simulink subsystem "decoder"  (R2019b)
settings: Solver=VariableStepAuto  StartTime=0.0  StopTime=10.0  RelTol=1e-3
InitFcn:
  | %% DSPBuilder Start
  | alt_dspbuilder_update_model(bdroot)
  | %% DSPBuilder End
StartFcn:
  | %% DSPBuilder Start
  | alt_dspbuilder_hdlimport_prepare_for_simulation(bdroot)
  | %% DSPBuilder End
undefined symbols (not defined in the file or in its folder): state
libraries: allblocks_alteradspbuilder2 x30
settings Model: Creator=vboxuser  LastModifiedBy=vboxuser

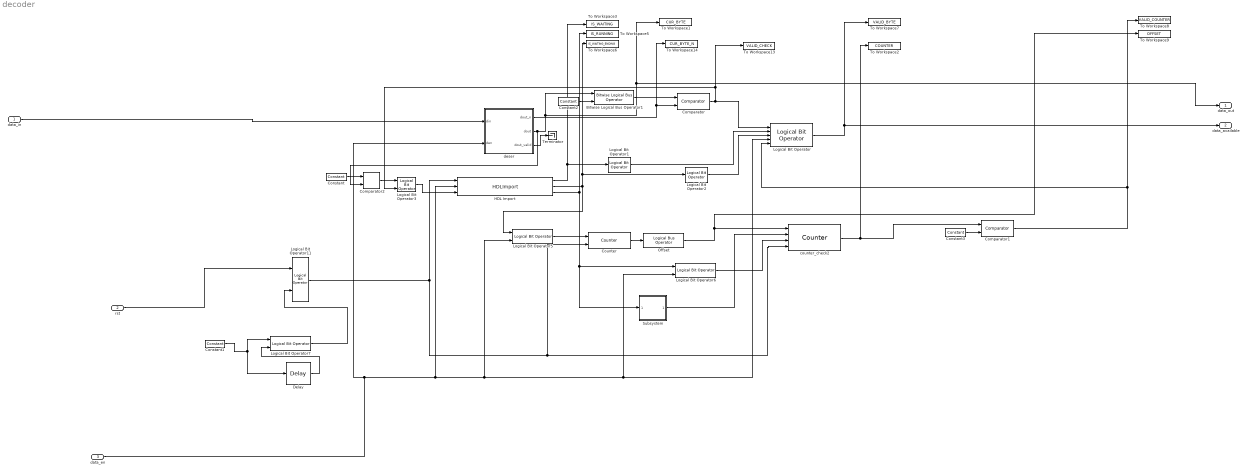
== system decoder ==
  data_in : Inport
  rst : Inport  Port=2
  data_en : Inport  Port=3
  Bitwise Logical Bus Operator1 : allblocks_alteradspbuilder2/Bitwise Logical Bus Operator  BusType=Unsigned Integer  bwl=8  bwr=0  LogicalOperator=XOR  pipeline_display=0
  Comparator : allblocks_alteradspbuilder2/Comparator  direction=a == b  pipeline_display=0  allowFloatingPointOverride=on  logOutputs=off  logFile=C:\Users\vboxuser\Documents\MATLAB\serializer\system2\tb_matcher_simu_old\matcher%5Fsimu%5Fold_Subsystem2_Subsystem_Comparator.fixedpointlog
  Comparator1 : allblocks_alteradspbuilder2/Comparator  direction=a == b  pipeline_display=0  allowFloatingPointOverride=on  logOutputs=off  logFile=C:\Users\vboxuser\Documents\MATLAB\serializer\system2\tb_matcher_simu_old\matcher%5Fsimu%5Fold_Subsystem2_Subsystem_Comparator1.fixedpointlog
  Comparator2 : allblocks_alteradspbuilder2/Comparator  direction=a == b  pipeline_display=0  allowFloatingPointOverride=on  logOutputs=off  logFile=C:\Users\vboxuser\Documents\MATLAB\serializer\system2\tb_matcher_simu_old\matcher%5Fsimu%5Fold_Subsystem2_Subsystem_Comparator2.fixedpointlog
  Constant : allblocks_alteradspbuilder2/Constant  mask_cst=71  BusType=Unsigned Integer  bwl=8  bwr=0  roundMode=Truncate  satMode=Wrap  SpecifyClock=off  allowFloatingPointOverride=on  logOutputs=off  logFile=C:\Users\vboxuser\Documents\MATLAB\serializer\system2\tb_matcher_simu_old\matcher%5Fsimu%5Fold_Subsystem2_Subsystem_Constant.fixedpointlog
  Constant1 : allblocks_alteradspbuilder2/Constant  mask_cst=1  BusType=Single Bit  bwl=8  bwr=0  roundMode=Truncate  satMode=Saturate  SpecifyClock=off  allowFloatingPointOverride=on  logOutputs=off  logFile=C:\Users\vboxuser\Documents\MATLAB\serializer\system2\tb_matcher_simu_old\matcher%5Fsimu%5Fold_Subsystem2_Subsystem_Constant1.fixedpointlog
  Constant2 : allblocks_alteradspbuilder2/Constant  mask_cst=255  BusType=Unsigned Integer  bwl=8  bwr=0  roundMode=Truncate  satMode=Wrap  SpecifyClock=off  allowFloatingPointOverride=on  logOutputs=off  logFile=C:\Users\vboxuser\Documents\MATLAB\serializer\system2\tb_matcher_simu_old\matcher%5Fsimu%5Fold_Subsystem2_Subsystem_Constant2.fixedpointlog
  Constant3 : allblocks_alteradspbuilder2/Constant  mask_cst=159  BusType=Unsigned Integer  bwl=8  bwr=0  roundMode=Truncate  satMode=Saturate  SpecifyClock=off  allowFloatingPointOverride=on  logOutputs=off  logFile=C:\Users\vboxuser\Documents\MATLAB\serializer\system2\tb_matcher_simu_old\matcher%5Fsimu%5Fold_Subsystem2_Subsystem_Constant3.fixedpointlog
  Counter : allblocks_alteradspbuilder2/Counter  BusType=Unsigned Integer  bwl=8  bwr=0  use_modulo=on  modulo=10  SpecifyClock=off  direction=Increment  use_sload=off  use_sset=off  svalue=1  use_clk_ena=off  use_ena=on  use_sclr=on  pipeline_display=1
  Delay : allblocks_alteradspbuilder2/Delay  pipeline=1  pipeline_display=1  ClockPhase=1  use_ena=off  use_sclr=off  allowFloatingPointOverride=on  logOutputs=off  logFile=C:\Users\vboxuser\Documents\MATLAB\serializer\system2\tb_matcher_simu_old\matcher%5Fsimu%5Fold_Subsystem2_Subsystem_Delay.fixedpointlog  use_init=off  reset_value=1
  HDL Import : allblocks_alteradspbuilder2/HDLImport  entityName=state_machine_import  inNames=rst ena is_matching  inBwls=1 1 1  inBwrs="0  0  0"  inTypes=b b b  inDelayed="0  0  0"  outNames=is_waiting is_waiting_ending is_running  outBwls=1 1 1  outBwrs="0  0  0"  outTypes=b b b  xmlmapfile=D:\pliki-programow\intel\18.1\quartus\dsp_builder\lib\SimgenCMap.xml  vofile=DSPBuilder_matcher_simu_import\state_machine.vo  src_file=state.v;  TopLevelName=state_machine  UseQPF=0  n_input_port=3  n_output_port=3  array_clocks=clk  use_systemC_model=off  is_megacore=off  use_dynamic_feedthrough_data=off  use_alphabetical_port_ordering=off  allowFloatingPointOverride=off  id=0  id_is_set=off  UseModelSimBasedFlow=off
  Logical Bit Operator : allblocks_alteradspbuilder2/Logical Bit Operator  LogicalOperator=AND  user_inputs=5  pipeline_display=0
  Logical Bit Operator1 : allblocks_alteradspbuilder2/Logical Bit Operator  LogicalOperator=NOT  user_inputs=2  pipeline_display=0
  Logical Bit Operator11 : allblocks_alteradspbuilder2/Logical Bit Operator  LogicalOperator=OR  user_inputs=2  pipeline_display=0
  Logical Bit Operator2 : allblocks_alteradspbuilder2/Logical Bit Operator  LogicalOperator=NOT  user_inputs=2  pipeline_display=0
  Logical Bit Operator3 : allblocks_alteradspbuilder2/Logical Bit Operator  LogicalOperator=AND  user_inputs=2  pipeline_display=0
  Logical Bit Operator5 : allblocks_alteradspbuilder2/Logical Bit Operator  LogicalOperator=AND  user_inputs=2  pipeline_display=0
  Logical Bit Operator6 : allblocks_alteradspbuilder2/Logical Bit Operator  LogicalOperator=AND  user_inputs=2  pipeline_display=0
  Logical Bit Operator7 : allblocks_alteradspbuilder2/Logical Bit Operator  LogicalOperator=XOR  user_inputs=2  pipeline_display=0
  Offset : allblocks_alteradspbuilder2/Logical Bus Operator  BusType=Unsigned Integer  bwl=8  bwr=0  LogicalOp_text=Shift Right  mask_value_num=-5  shift_amount=1  force_sign_ext=on  pipeline_display=0
  Subsystem : Subsystem  ReferencedSubsystem=Puls
  Terminator : Terminator
  To Workspace1 : ToWorkspace  VariableName=CUR_BYTE  SampleTime=-1
      settings: Save2DSignal=2-D array (concatenate along first dimension)
  To Workspace13 : ToWorkspace  VariableName=VALID_CHECK  SampleTime=-1
      settings: Save2DSignal=2-D array (concatenate along first dimension)
  To Workspace14 : ToWorkspace  VariableName=CUR_BYTE_N  SampleTime=-1
      settings: Save2DSignal=2-D array (concatenate along first dimension)
  To Workspace2 : ToWorkspace  VariableName=COUNTER  SampleTime=-1
      settings: Save2DSignal=2-D array (concatenate along first dimension)
  To Workspace3 : ToWorkspace  VariableName=IS_WAITING  SampleTime=-1
      settings: Save2DSignal=2-D array (concatenate along first dimension)
  To Workspace5 : ToWorkspace  VariableName=IS_RUNNING  SampleTime=-1
      settings: Save2DSignal=2-D array (concatenate along first dimension)
  To Workspace6 : ToWorkspace  VariableName=IS_WAITING_ENDING  SampleTime=-1
      settings: Save2DSignal=2-D array (concatenate along first dimension)
  To Workspace7 : ToWorkspace  VariableName=VALID_BYTE  SampleTime=-1
      settings: Save2DSignal=2-D array (concatenate along first dimension)
  To Workspace8 : ToWorkspace  VariableName=VALID_COUNTER  SampleTime=-1
      settings: Save2DSignal=2-D array (concatenate along first dimension)
  To Workspace9 : ToWorkspace  VariableName=OFFSET  SampleTime=-1
      settings: Save2DSignal=2-D array (concatenate along first dimension)
  counter_check2 : allblocks_alteradspbuilder2/Counter  BusType=Unsigned Integer  bwl=8  bwr=0  use_modulo=on  modulo=160  SpecifyClock=off  direction=Increment  use_sload=on  use_sset=off  svalue=1  use_clk_ena=off  use_ena=on  use_sclr=on  pipeline_display=1
  deser : Subsystem
  data_out : Outport
  data_available : Outport  Port=2
  wires:
  Subsystem/1 -> counter_check2/2
  rst/1 -> Logical Bit Operator11/1
  data_in/1 -> deser/1(din)
  Logical Bit Operator11/1 -> Counter/2, counter_check2/4, HDL Import/1
  deser/3(dout_valid) -> Terminator/1
  Logical Bit Operator7/1 -> Logical Bit Operator11/2
  Delay/1 -> Logical Bit Operator7/2
  Constant1/1 -> Logical Bit Operator7/1, Delay/1
  Logical Bit Operator6/1 -> counter_check2/3
  Counter/1 -> Offset/1
  Constant2/1 -> Bitwise Logical Bus Operator1/2
  Bitwise Logical Bus Operator1/1 -> Comparator/1
  Offset/1 -> To Workspace9/1, counter_check2/1
  Logical Bit Operator1/1 -> Logical Bit Operator/2
  Logical Bit Operator/1 -> data_available/1, To Workspace7/1
  HDL Import/1 -> To Workspace3/1, Logical Bit Operator1/1
  Constant3/1 -> Comparator1/2
  Comparator/1 -> Logical Bit Operator/1, To Workspace13/1, Logical Bit Operator3/2
  HDL Import/3 -> Subsystem/1, Logical Bit Operator6/1, To Workspace5/1
  Comparator1/1 -> Logical Bit Operator/5, To Workspace8/1
  deser/2(dout) -> data_out/1, To Workspace1/1, Bitwise Logical Bus Operator1/1, Comparator2/2
  Logical Bit Operator3/1 -> HDL Import/3
  deser/1(dout_n) -> To Workspace14/1, Comparator/2
  HDL Import/2 -> To Workspace6/1, Logical Bit Operator2/1, Logical Bit Operator5/1
  data_en/1 -> Logical Bit Operator5/2, Logical Bit Operator6/2, Logical Bit Operator/4, HDL Import/2, deser/2(den)
  counter_check2/1 -> To Workspace2/1, Comparator1/1
  Logical Bit Operator2/1 -> Logical Bit Operator/3
  Logical Bit Operator5/1 -> Counter/1
  Constant/1 -> Comparator2/1
  Comparator2/1 -> Logical Bit Operator3/1

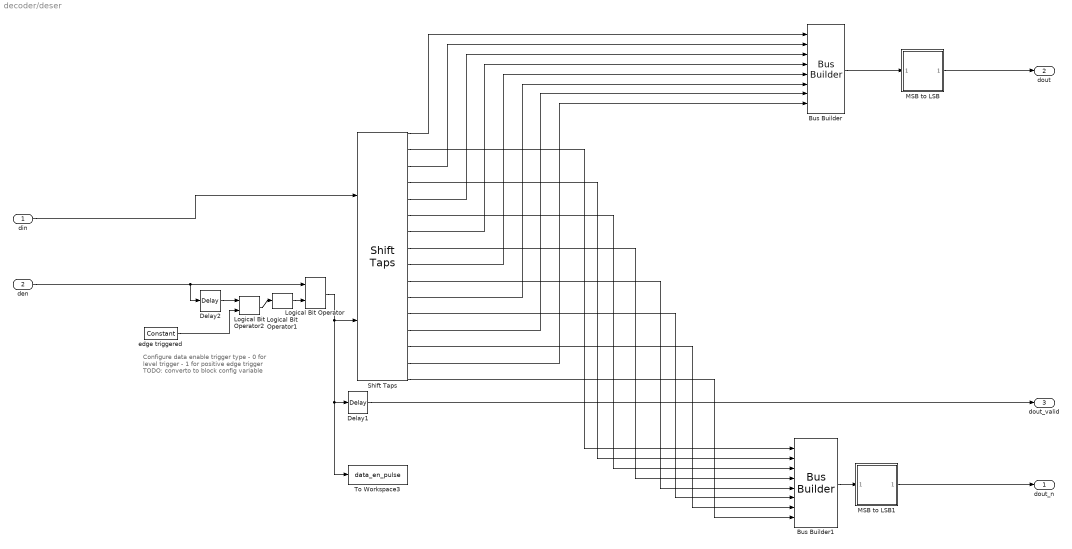
== system decoder/deser ==
  note: Configure data enable trigger type
      |  - 0 for level trigger
      |  - 1 for positive edge trigger
      |
      | TODO: converto to block config variable
  din : Inport
  den : Inport  Port=2
  Bus Builder : allblocks_alteradspbuilder2/Bus Builder  BusType=Unsigned Integer  bwl=8  bwr=1  pipeline_display=0
  Bus Builder1 : allblocks_alteradspbuilder2/Bus Builder  BusType=Unsigned Integer  bwl=8  bwr=1  pipeline_display=0
  Delay1 : allblocks_alteradspbuilder2/Delay  pipeline=1  pipeline_display=1  ClockPhase=1  use_ena=off  use_sclr=off  allowFloatingPointOverride=on  logOutputs=off  logFile=C:\Users\vboxuser\Documents\MATLAB\serializer\system2\tb_matcher_simu_old\matcher%5Fsimu%5Fold_Subsystem2_Subsystem_deser_Delay1.fixedpointlog  use_init=off  reset_value=1
  Delay2 : allblocks_alteradspbuilder2/Delay  pipeline=1  pipeline_display=1  ClockPhase=1  use_ena=off  use_sclr=off  allowFloatingPointOverride=on  logOutputs=off  logFile=C:\Users\vboxuser\Documents\MATLAB\serializer\system2\tb_matcher_simu_old\matcher%5Fsimu%5Fold_Subsystem2_Subsystem_deser_Delay2.fixedpointlog  use_init=off  reset_value=1
  Logical Bit Operator : allblocks_alteradspbuilder2/Logical Bit Operator  LogicalOperator=AND  user_inputs=2  pipeline_display=0
  Logical Bit Operator1 : allblocks_alteradspbuilder2/Logical Bit Operator  LogicalOperator=NOT  user_inputs=2  pipeline_display=0
  Logical Bit Operator2 : allblocks_alteradspbuilder2/Logical Bit Operator  LogicalOperator=AND  user_inputs=2  pipeline_display=0
  MSB to LSB : Subsystem  ReferencedSubsystem=MSB_to_LSB
  MSB to LSB1 : Subsystem  ReferencedSubsystem=MSB_to_LSB
  Shift Taps : allblocks_alteradspbuilder2/Shift Taps  number_of_taps=16  tap_distance=10  use_shiftout=off  use_ena=on  use_sclr=off  use_dedicated_circuitry=on  ram_type=AUTO  allowFloatingPointOverride=on  logOutputs=off  logFile=C:\Users\vboxuser\Documents\MATLAB\serializer\system2\tb_matcher_simu_old\matcher%5Fsimu%5Fold_Subsystem2_Subsystem_deser_Shift+Taps%3A%3At.fixedpointlog,C:\Users\vboxuser\Documents\MATLAB\serializer\system2\tb_matcher_simu_old\matcher%5Fsimu%5Fold_Subsystem2_Subsystem_deser_Shift+Taps%3A%3At.fixedpointlog,C:\Users\vboxuser\Documents\MATLAB\serializer\system2\tb_matcher_simu_old\matcher%5Fsimu%5Fold_Subsystem2_Subsystem_deser_Shift+Taps%3A%3At.fixedpointlog,C:\Users\vboxuser\Documents\MATLAB\serializer\system2\tb_matcher_simu_old\matcher%5Fsimu%5Fold_Subsystem2_Subsystem_deser_Shift+Taps%3A%3At.fixedpointlog,C:\Users\vboxuser\Documents\MATLAB\serializer\system2\tb_matcher_simu_old\matcher%5Fsimu%5Fold_Subsystem2_Subsystem_deser_Shift+Taps%3A%3At.fixedpointlog,C:\Users\vboxuser\Documents\MATLAB\serializer\system2\tb_matcher_simu_old\matcher%5Fsimu%5Fold_Subsystem2_Subsystem_deser_Shift+Taps%3A%3At.fixedpointlog,C:\Users\vboxuser\Documents\MATLAB\serializer\system2\tb_matcher_simu_old\matcher%5Fsimu%5Fold_Subsystem2_Subsystem_deser_Shift+Taps%3A%3At.fixedpointlog,C:\Users\vboxuser\Documents\MATLAB\serializer\system2\tb_matcher_simu_old\matcher%5Fsimu%5Fold_Subsystem2_Subsystem_deser_Shift+Taps%3A%3At.fixedpointlog,C:\Users\vboxuser\Documents\MATLAB\serializer\system2\tb_matcher_simu_old\matcher%5Fsimu%5Fold_Subsystem2_Subsystem_deser_Shift+Taps%3A%3At.fixedpointlog,C:\Users\vboxuser\Documents\MATLAB\serializer\system2\tb_matcher_simu_old\matcher%5Fsimu%5Fold_Subsystem2_Subsystem_deser_Shift+Taps%3A%3At.fixedpointlog,C:\Users\vboxuser\Documents\MATLAB\serializer\system2\tb_matcher_simu_old\matcher%5Fsimu%5Fold_Subsystem2_Subsystem_deser_Shift+Taps%3A%3At.fixedpointlog,C:\Users\vboxuser\Documents\MATLAB\serializer\system2\tb_matcher_simu_old\matcher%5Fsimu%5Fold_Subsystem2_Subsystem_deser_Shift+Taps%3A%3At.fixedpointlog,C:\Users\vboxuser\Documents\MATLAB\serializer\system2\tb_matcher_simu_old\matcher%5Fsimu%5Fold_Subsystem2_Subsystem_deser_Shift+Taps%3A%3At.fixedpointlog,C:\Users\vboxuser\Documents\MATLAB\serializer\system2\tb_matcher_simu_old\matcher%5Fsimu%5Fold_Subsystem2_Subsystem_deser_Shift+Taps%3A%3At.fixedpointlog,C:\Users\vboxuser\Documents\MATLAB\serializer\system2\tb_matcher_simu_old\matcher%5Fsimu%5Fold_Subsystem2_Subsystem_deser_Shift+Taps%3A%3At.fixedpointlog,C:\Users\vboxuser\Documents\MATLAB\serializer\system2\tb_matcher_simu_old\matcher%5Fsimu%5Fold_Subsystem2_Subsystem_deser_Shift+Taps%3A%3At.fixedpointlog,
  To Workspace3 : ToWorkspace  VariableName=data_en_pulse  SampleTime=-1
      settings: Save2DSignal=2-D array (concatenate along first dimension)
  edge triggered : allblocks_alteradspbuilder2/Constant  mask_cst=0  BusType=Single Bit  bwl=8  bwr=0  roundMode=Truncate  satMode=Wrap  SpecifyClock=off  allowFloatingPointOverride=on  logOutputs=off  logFile=C:\Users\vboxuser\Documents\MATLAB\serializer\system2\tb_matcher_simu_old\matcher%5Fsimu%5Fold_Subsystem2_Subsystem_deser_edge+triggered.fixedpointlog
  dout_n : Outport
  dout : Outport  Port=2
  dout_valid : Outport  Port=3
  wires:
  din/1 -> Shift Taps/1
  MSB to LSB/1 -> dout/1
  edge triggered/1 -> Logical Bit Operator2/2
  MSB to LSB1/1 -> dout_n/1
  Shift Taps/8 -> Bus Builder1/4
  den/1 -> Logical Bit Operator/1, Delay2/1
  Logical Bit Operator1/1 -> Logical Bit Operator/2
  Shift Taps/12 -> Bus Builder1/6
  Shift Taps/7 -> Bus Builder/4
  Logical Bit Operator/1 -> Shift Taps/2, To Workspace3/1, Delay1/1
  Shift Taps/10 -> Bus Builder1/5
  Shift Taps/14 -> Bus Builder1/7
  Delay1/1 -> dout_valid/1
  Shift Taps/1 -> Bus Builder/1
  Logical Bit Operator2/1 -> Logical Bit Operator1/1
  Shift Taps/13 -> Bus Builder/7
  Shift Taps/9 -> Bus Builder/5
  Shift Taps/15 -> Bus Builder/8
  Bus Builder1/1 -> MSB to LSB1/1
  Shift Taps/11 -> Bus Builder/6
  Shift Taps/16 -> Bus Builder1/8
  Shift Taps/4 -> Bus Builder1/2
  Delay2/1 -> Logical Bit Operator2/1
  Shift Taps/3 -> Bus Builder/2
  Shift Taps/2 -> Bus Builder1/1
  Bus Builder/1 -> MSB to LSB/1
  Shift Taps/5 -> Bus Builder/3
  Shift Taps/6 -> Bus Builder1/3
